simulink model "respuesta_segundo_orden"  (R2025b)
settings: Solver=FixedStepDiscrete  StartTime=0.0  StopTime=inf  FixedStep=1e-4  MaxStep=1/10000  RelTol=1e-3
StopFcn:
  | daqreset
settings Model: Creator=jesus  LastModifiedBy=jesus

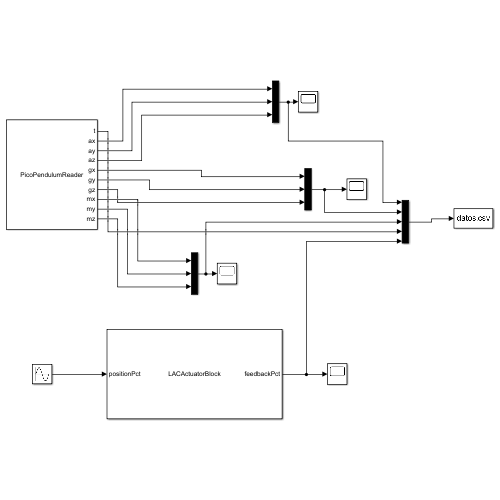
[thumbnail: Simulink's stored preview of the top-level diagram]
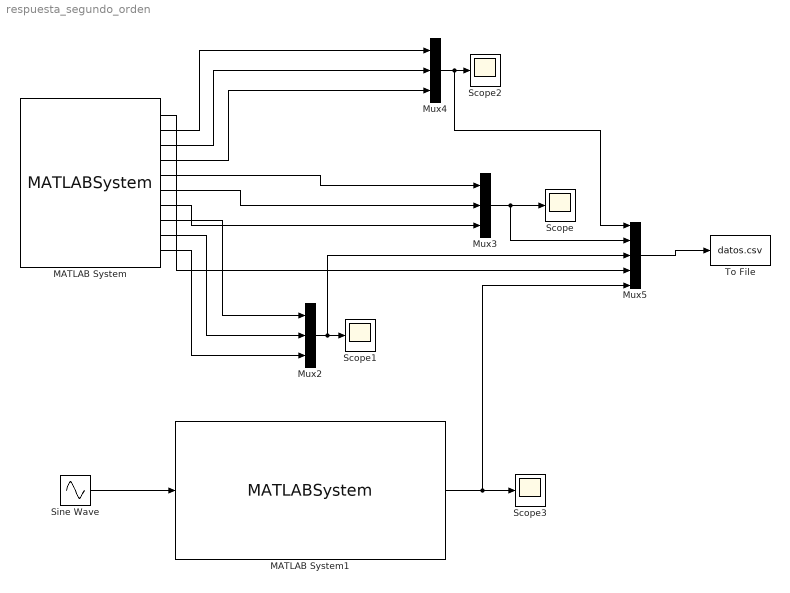
== system respuesta_segundo_orden ==
  MATLAB System : MATLABSystem  System=PicoPendulumReader  Host=192.168.1.118  Port=4242  Rate=200  Timeout=5  StartOnSetup=true
      mask Type: PicoPendulumReader
  MATLAB System1 : MATLABSystem  System=LACActuatorBlock  Rate=50  StrokeMM=50  VID=uint16(0)  PID=uint16(0)  RetractOnStop=true
      mask Type: LACActuatorBlock
  Mux2 : Mux  Inputs=3
  Mux3 : Mux  Inputs=3
  Mux4 : Mux  Inputs=3
  Mux5 : Mux  Inputs=5
  Scope{,1..3} (4 alike) : Scope
      Scope settings: ActiveDisplayYMinimum=-39.32824475  ActiveDisplayYMaximum=35.17557275
      Scope1 settings: ActiveDisplayYMinimum=-96.5392217532128  ActiveDisplayYMaximum=94.789638652650652
      Scope2 settings: DataLoggingVariableName=ScopeData2
      Scope3 settings: ActiveDisplayYMinimum=-96.5392217532128  ActiveDisplayYMaximum=94.789638652650652  DataLoggingVariableName=ScopeData3
  Sine Wave : Sin  Amplitude=10  Bias=60  Frequency=2*pi*10  SampleTime=0
  To File : ToFile  Filename=datos.csv  MatrixName=senales
  wires:
  Mux5/1 -> To File/1
  Mux3/1 -> Mux5/2, Scope/1
  Mux2/1 -> Mux5/3, Scope1/1
  MATLAB System/8 -> Mux2/1
  MATLAB System/9 -> Mux2/2
  MATLAB System/10 -> Mux2/3
  MATLAB System/2 -> Mux4/1
  MATLAB System/3 -> Mux4/2
  MATLAB System/4 -> Mux4/3
  Mux4/1 -> Mux5/1, Scope2/1
  MATLAB System/5 -> Mux3/1
  MATLAB System/6 -> Mux3/2
  MATLAB System/7 -> Mux3/3
  MATLAB System/1 -> Mux5/4
  Sine Wave/1 -> MATLAB System1/1
  MATLAB System1/1 -> Mux5/5, Scope3/1
